simulink model "Concrete_Mix_Design_Simulink_v9"  (R2020a)
settings: Solver=VariableStepAuto  StartTime=0.0  StopTime=10.0  RelTol=1e-3
settings Model: Creator=SMONE  LastModifiedBy=SMONE

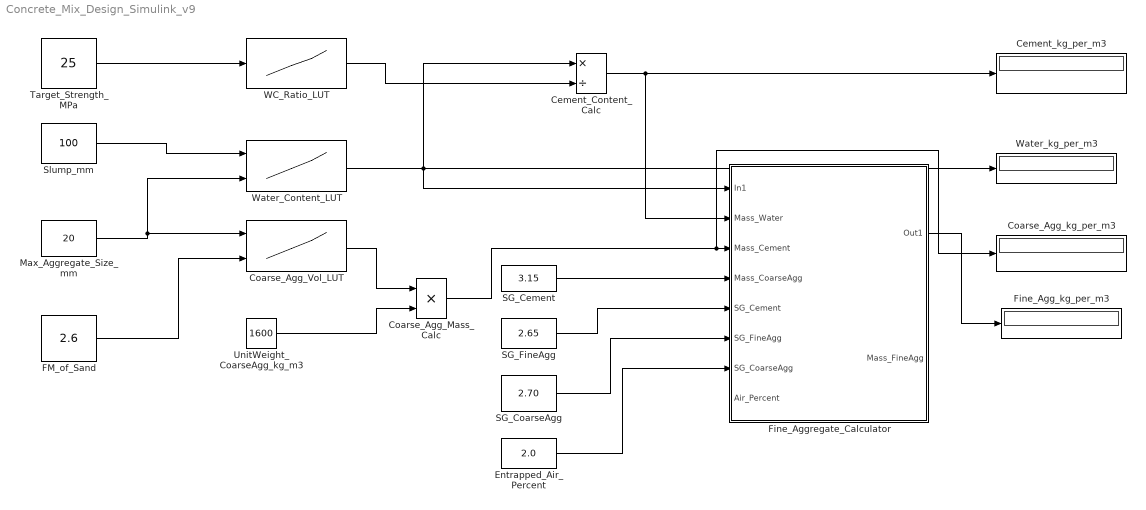
== system Concrete_Mix_Design_Simulink_v9 ==
  Cement_Content_Calc : Product  Inputs=*/
  Cement_kg_per_m3 : Display
  Coarse_Agg_Mass_Calc : Product
  Coarse_Agg_Vol_LUT : Lookup_n-D  BreakpointsForDimension1=[10 20 40]  BreakpointsForDimension2=[2.4 2.6 2.8]  Table=[0.5 0.48 0.46;0.66 0.64 0.62;0.75 0.73 0.71]  InternalRulePriority=Speed  RndMeth=Simplest  InputSameDT=on
  Coarse_Agg_kg_per_m3 : Display
  Entrapped_Air_Percent : Constant  Value=2.0
  FM_of_Sand : Constant  Value=2.6
  Fine_Agg_kg_per_m3 : Display
  Fine_Aggregate_Calculator : Subsystem
  Max_Aggregate_Size_mm : Constant  Value=20
  SG_Cement : Constant  Value=3.15
  SG_CoarseAgg : Constant  Value=2.70
  SG_FineAgg : Constant  Value=2.65
  Slump_mm : Constant  Value=100
  Target_Strength_MPa : Constant  Value=25
  UnitWeight_CoarseAgg_kg_m3 : Constant  Value=1600
  WC_Ratio_LUT : Lookup_n-D  NumberOfTableDimensions=1  BreakpointsForDimension1=[25 35 45]  Table=[0.65 0.52 0.42]  InternalRulePriority=Speed  RndMeth=Simplest  InputSameDT=on
  Water_Content_LUT : Lookup_n-D  BreakpointsForDimension1=[37.5 87.5]  BreakpointsForDimension2=[10 20 40]  Table=[215 190 175;225 205 185]  InternalRulePriority=Speed  RndMeth=Simplest  InputSameDT=on
  Water_kg_per_m3 : Display
  wires:
  Fine_Aggregate_Calculator/1(Out1) -> Fine_Agg_kg_per_m3/1
  SG_FineAgg/1 -> Fine_Aggregate_Calculator/5(SG_Cement)
  Entrapped_Air_Percent/1 -> Fine_Aggregate_Calculator/7(SG_CoarseAgg)
  Coarse_Agg_Vol_LUT/1 -> Coarse_Agg_Mass_Calc/1
  SG_CoarseAgg/1 -> Fine_Aggregate_Calculator/6(SG_FineAgg)
  SG_Cement/1 -> Fine_Aggregate_Calculator/4(Mass_CoarseAgg)
  WC_Ratio_LUT/1 -> Cement_Content_Calc/2
  UnitWeight_CoarseAgg_kg_m3/1 -> Coarse_Agg_Mass_Calc/2
  FM_of_Sand/1 -> Coarse_Agg_Vol_LUT/2
  Target_Strength_MPa/1 -> WC_Ratio_LUT/1
  Slump_mm/1 -> Water_Content_LUT/1
  Coarse_Agg_Mass_Calc/1 -> Coarse_Agg_kg_per_m3/1, Fine_Aggregate_Calculator/3(Mass_Cement)
  Cement_Content_Calc/1 -> Fine_Aggregate_Calculator/2(Mass_Water), Cement_kg_per_m3/1
  Water_Content_LUT/1 -> Cement_Content_Calc/1, Fine_Aggregate_Calculator/1(In1), Water_kg_per_m3/1
  Max_Aggregate_Size_mm/1 -> Water_Content_LUT/2, Coarse_Agg_Vol_LUT/1

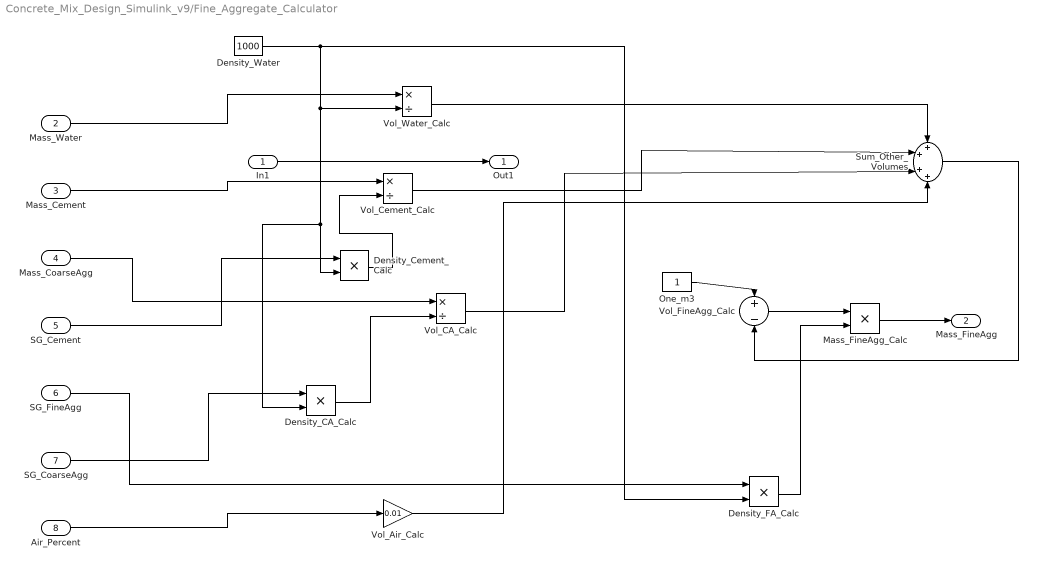
== system Concrete_Mix_Design_Simulink_v9/Fine_Aggregate_Calculator ==
  In1 : Inport
  Mass_Water : Inport  Port=2
  Mass_Cement : Inport  Port=3
  Mass_CoarseAgg : Inport  Port=4
  SG_Cement : Inport  Port=5
  SG_FineAgg : Inport  Port=6
  SG_CoarseAgg : Inport  Port=7
  Air_Percent : Inport  Port=8
  Density_CA_Calc : Product  Inputs=**
  Density_Cement_Calc : Product  Inputs=**
  Density_FA_Calc : Product  Inputs=**
  Density_Water : Constant  Value=1000
  Mass_FineAgg_Calc : Product  Inputs=**
  One_m3 : Constant
  Sum_Other_Volumes : Sum  Inputs=++++
  Vol_Air_Calc : Gain  Gain=0.01
  Vol_CA_Calc : Product  Inputs=*/
  Vol_Cement_Calc : Product  Inputs=*/
  Vol_FineAgg_Calc : Sum  Inputs=+-
  Vol_Water_Calc : Product  Inputs=*/
  Out1 : Outport
  Mass_FineAgg : Outport  Port=2
  wires:
  In1/1 -> Out1/1
  Mass_Water/1 -> Vol_Water_Calc/1
  Density_Water/1 -> Density_Cement_Calc/2, Density_CA_Calc/2, Vol_Water_Calc/2, Density_FA_Calc/2
  SG_Cement/1 -> Density_Cement_Calc/1
  Mass_Cement/1 -> Vol_Cement_Calc/1
  Density_Cement_Calc/1 -> Vol_Cement_Calc/2
  SG_CoarseAgg/1 -> Density_CA_Calc/1
  Mass_CoarseAgg/1 -> Vol_CA_Calc/1
  Density_CA_Calc/1 -> Vol_CA_Calc/2
  Air_Percent/1 -> Vol_Air_Calc/1
  Vol_Water_Calc/1 -> Sum_Other_Volumes/1
  Vol_Cement_Calc/1 -> Sum_Other_Volumes/2
  Vol_CA_Calc/1 -> Sum_Other_Volumes/3
  Vol_Air_Calc/1 -> Sum_Other_Volumes/4
  One_m3/1 -> Vol_FineAgg_Calc/1
  Sum_Other_Volumes/1 -> Vol_FineAgg_Calc/2
  SG_FineAgg/1 -> Density_FA_Calc/1
  Vol_FineAgg_Calc/1 -> Mass_FineAgg_Calc/1
  Density_FA_Calc/1 -> Mass_FineAgg_Calc/2
  Mass_FineAgg_Calc/1 -> Mass_FineAgg/1
